simulink model "MotorSpeedModelingSimscape"  (R2015b)
settings: Solver=VariableStepAuto  StartTime=0.0  StopTime=10.0  RelTol=1e-3
values from neighbouring files (symbols this model uses):
  b = str2num(get(handles.frictionText,'String'))    [MotorSpeedControlSimulink.m]    (also in MotorSpeedSimscapeModeling.m = str2num(get(handles.dampingText,'String')))
  K = str2num(get(handles.emfText,'String'))    [MotorSpeedSimscapeModeling.m]
  R = str2num(get(handles.resistanceText,'String'))    [MotorSpeedControlSimulink.m]    (also in MotorSpeedSimscapeModeling.m)
libraries: fl_lib x10, nesl_utility x5
settings Model: Creator=YOUNG  LastModifiedBy=YOUNG

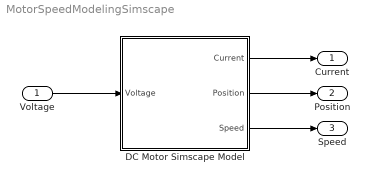
== system MotorSpeedModelingSimscape ==
  Voltage : Inport
  DC Motor Simscape Model : Subsystem
      mask Display: image(imread('dc_motor_diagram.jpg'));
  Current : Outport
  Position : Outport  Port=2
  Speed : Outport  Port=3
  wires:
  Voltage/1 -> DC Motor Simscape Model/1(Voltage)
  DC Motor Simscape Model/1(Current) -> Current/1
  DC Motor Simscape Model/2(Position) -> Position/1
  DC Motor Simscape Model/3(Speed) -> Speed/1

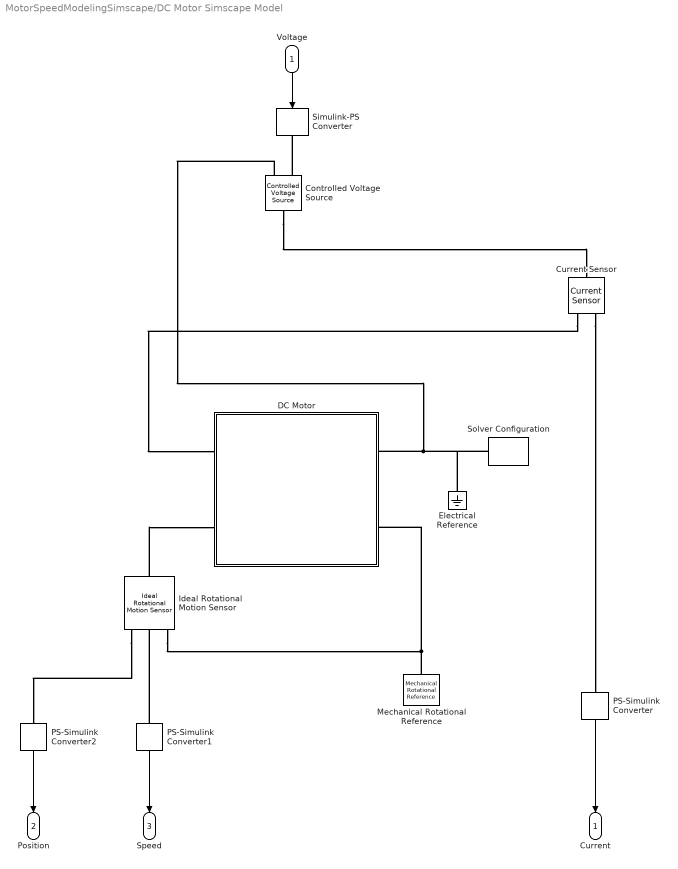
== system MotorSpeedModelingSimscape/DC Motor Simscape Model ==
  Voltage : Inport
  Controlled Voltage Source : fl_lib/Electrical/Electrical Sources/Controlled Voltage Source
  Current Sensor : fl_lib/Electrical/Electrical Sensors/Current Sensor
  DC Motor : Subsystem
      mask Display: image(imread('Electric_motor_cycle_2.jpg'));
  Electrical Reference : fl_lib/Electrical/Electrical Elements/Electrical Reference
  Ideal Rotational Motion Sensor : fl_lib/Mechanical/Mechanical Sensors/Ideal Rotational Motion Sensor  offset=0 rad
  Mechanical Rotational Reference : fl_lib/Mechanical/Rotational Elements/Mechanical Rotational Reference
  PS-Simulink Converter : nesl_utility/PS-Simulink Converter  PhysicalDomain=network_engine_domain  SubClassName=ps_output  LeftPortType=input  RightPortType=output  PseudoPeriodic=off  Frequencies=[]  Unit=1  AffineConversion=off
  PS-Simulink Converter1 : nesl_utility/PS-Simulink Converter  PhysicalDomain=network_engine_domain  SubClassName=ps_output  LeftPortType=input  RightPortType=output  PseudoPeriodic=off  Frequencies=[]  Unit=1  AffineConversion=off
  PS-Simulink Converter2 : nesl_utility/PS-Simulink Converter  PhysicalDomain=network_engine_domain  SubClassName=ps_output  LeftPortType=input  RightPortType=output  PseudoPeriodic=off  Frequencies=[]  Unit=1  AffineConversion=off
  Simulink-PS Converter : nesl_utility/Simulink-PS Converter  PhysicalDomain=network_engine_domain  SubClassName=ps_input  LeftPortType=input  RightPortType=output  PseudoPeriodic=off  Frequencies=[]  NoiseDistribution=none  NoiseParameters=[]  Unit=1  AffineConversion=off  InputFiltering=off  SimscapeFilterOrder=1  InputFilterTimeConstant=0.001  UdotUserProvided=1
  Solver Configuration : nesl_utility/Solver Configuration  PhysicalDomain=network_engine_domain  SubClassName=solver  LeftPortType=input  RightPortType=generic  Accelerate=off  Tones=[]  Harmonics=[]  SimulateNoise=off  Profile=off  UseLocalSampling=off  EnableSwitchedLinearOptims=on  FrequencyDomain=off  UseCCode=off  RelTol=0.001  AbsTol=1e-06  MinStep=1e-09  ToWorkspace=off  RevertToSquareIcSolve=off  NumHomotopyIterations=100  PhasorMode=off  PhasorModeNumHarmonics=1  DoDC=off  ResidualTolerance=1e-09  UseLocalSolver=off  LocalSolverChoice=NE_BACKWARD_EULER_ADVANCER  LocalSolverSampleTime=0.001  DoFixedCost=off  MaxNonlinIter=3  MaxModeIter=2  LinearAlgebra=Sparse  DelaysMemoryBudget=1024  AutomaticFiltering=on  FilteringTimeConstant=0.001
  Current : Outport
  Position : Outport  Port=2
  Speed : Outport  Port=3
  wires:
  PS-Simulink Converter2/1 -> Position/1
  PS-Simulink Converter/1 -> Current/1
  Voltage/1 -> Simulink-PS Converter/1
  PS-Simulink Converter1/1 -> Speed/1
  connections:
  Controlled Voltage Source/LConn1 -- Current Sensor/LConn1
  PS-Simulink Converter1/LConn1 -- Ideal Rotational Motion Sensor/RConn2
  Ideal Rotational Motion Sensor/LConn1 -- DC Motor/LConn2
  Current Sensor/RConn2 -- DC Motor/LConn1
  Controlled Voltage Source/RConn1 -- Simulink-PS Converter/RConn1
  Controlled Voltage Source/RConn2 -- Electrical Reference/LConn1 -- Solver Configuration/RConn1 -- DC Motor/RConn1
  Ideal Rotational Motion Sensor/RConn3 -- PS-Simulink Converter2/LConn1
  Mechanical Rotational Reference/LConn1 -- Ideal Rotational Motion Sensor/RConn1 -- DC Motor/RConn2
  Current Sensor/RConn1 -- PS-Simulink Converter/LConn1

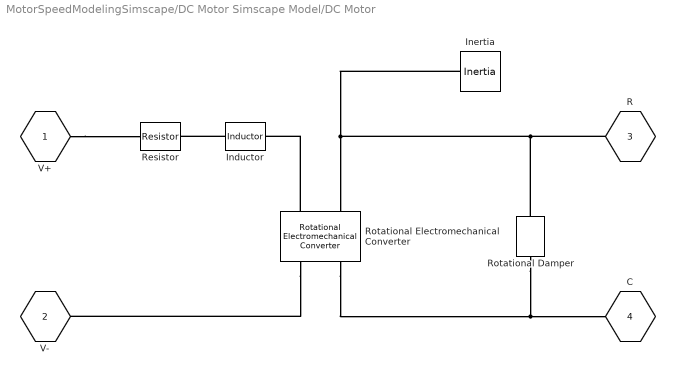
== system MotorSpeedModelingSimscape/DC Motor Simscape Model/DC Motor ==
  Inductor : fl_lib/Electrical/Electrical Elements/Inductor  l=L H  r=0 Ohm  g=1e-9 1/Ohm  i_specify=off  i_priority=None  i=0 A  v_specify=off  v_priority=None  v=0 V  i_L_specify=off  i_L_priority=None  i_L=0 A
  Inertia : fl_lib/Mechanical/Rotational Elements/Inertia  inertia=J kg*m^2  w_specify=off  w_priority=None  w=0 rad/s  t_specify=off  t_priority=None  t=0 N*m
  Resistor : fl_lib/Electrical/Electrical Elements/Resistor  R=R Ohm  i_specify=off  i_priority=None  i=0 A  v_specify=off  v_priority=None  v=0 V
  Rotational Electromechanical Converter : fl_lib/Electrical/Electrical Elements/Rotational Electromechanical Converter  K=K V/(rad/s)  i_specify=off  i_priority=None  i=0 A  v_specify=off  v_priority=None  v=0 V  t_specify=off  t_priority=None  t=0 N*m  w_specify=off  w_priority=None  w=0 rad/s
  Rotational Damper : fl_lib/Mechanical/Rotational Elements/Rotational Damper  D=b N*m/(rad/s)  w_specify=off  w_priority=None  w=0 rad/s  t_specify=off  t_priority=None  t=0 N*m
  V+ : PMIOPort  Port=1  Side=Left
  V- : PMIOPort  Port=2  Side=Right
  R : PMIOPort  Port=3  Side=Left
  C : PMIOPort  Port=4  Side=Right
  connections:
  Inductor/LConn1 -- Resistor/RConn1
  Rotational Electromechanical Converter/RConn1 -- V-/RConn1
  Rotational Electromechanical Converter/LConn1 -- Inductor/RConn1
  Inertia/LConn1 -- Rotational Electromechanical Converter/LConn2 -- R/RConn1 -- Rotational Damper/RConn1
  Rotational Electromechanical Converter/RConn2 -- C/RConn1 -- Rotational Damper/LConn1
  V+/RConn1 -- Resistor/LConn1
